simulink model "rtwdemo_sil_counter"  (Simulink 7.6)
settings: Solver=FixedStepDiscrete  StartTime=0.0  StopTime=10.0  FixedStep=Auto  RelTol=1e-3  SampleTimeConstraint=STIndependent
model workspace (MAT data in the model file):
  myUpper : Simulink.Parameter (value not decoded)
  myLower : Simulink.Parameter (value not decoded)
PostLoadFcn:
  | rtwdemo_overrides='{''SupportAbsoluteTime'',''LaunchReport'',''PassReuseOutputArgsAs''}';
  | rtwconfiguredemo(gcs,'noop',false,rtwdemo_overrides);
  | rtwdemo_cs=getActiveConfigSet(gcs);
  | setProp(rtwdemo_cs,'CustomSymbolStr','$R$N$M');
  | set_param(gcs,'dirty','off');
  | clear rtwdemo_overrides rtwdemo_cs
  | 
  | rtwdemo_sil_modelblock_data
undefined symbols (not defined in the file or in its folder): Increment
Description:
  | Example model reference component.
settings Model: Creator=The MathWorks Inc.  ExtModeAutoUpdateStatusClock=off
settings DataIOCC: LimitDataPoints=off  SaveFormat=StructureWithTime  SaveOutput=off  SaveTime=off  SignalLoggingName=logsOut
settings OptimizationCC: InlineParams=on  UseIntDivNetSlope=on  InlineInvariantSignals=on  EnhancedBackFolding=on  BooleansAsBitfields=on  PassReuseOutputArgsAs=Individual arguments  StateBitsets=on  DataBitsets=on  UseTempVars=on  ZeroExternalMemoryAtStartup=off  ZeroInternalMemoryAtStartup=off  NoFixptDivByZeroProtection=on  EfficientFloat2IntCast=on  OptimizeModelRefInitCode=on  LifeSpan=1  SimCompilerOptimization=On
settings DebuggingCC: MergeDetectMultiDrivingBlocksExec=error  CheckExecutionContextPreStartOutputMsg=on  CheckExecutionContextRuntimeOutputMsg=on  SolverPrmCheckMsg=none  UniqueDataStoreMsg=error  ModelReferenceSymbolNameMessage=none  StrictBusMsg=ErrorOnBusTreatedAsVector
settings HardwareCC: ProdIntDivRoundTo=Zero  ProdEndianess=LittleEndian  ProdHWDeviceType=Specified  TargetHWDeviceType=Generic->32-bit Embedded Processor
settings ModelReferenceCC: CheckModelReferenceTargetMessage=none  ModelReferencePassRootInputsByReference=off
settings RTWCC: SystemTargetFile=ert.tlc  TLCOptions=-p0 -aWarnNonSaturatedBlocks=0  TemplateMakefile=ert_default_tmf  Description=Real-Time Workshop Embedded Coder  GenerateReport=on  RTWVerbose=off  ProcessScript=ert_make_rtw_hook  IncludeHyperlinkInReport=on  GenerateTraceInfo=on  GenerateTraceReport=on  GenerateTraceReportSl=on  GenerateTraceReportSf=on  GenerateTraceReportEml=on
settings CodeAppCC: ForceParamTrailComments=on  IgnoreCustomStorageClasses=off  IgnoreTestpoints=on  SimulinkDataObjDesc=on  CustomSymbolStrGlobalVar=rt$N$M  CustomSymbolStrType=$N$M  CustomSymbolStrFcn=$N$M$F  CustomSymbolStrMacro=$N$M  InsertBlockDesc=on
settings ERTTargetCC: MultiwordLength=2048  GenerateSampleERTMain=on  IncludeMdlTerminateFcn=off  CombineSignalStateStructs=on  SupportAbsoluteTime=off  SupportNonFinite=off  SupportComplex=off  InlinedParameterPlacement=NonHierarchical  ERTCustomFileTemplate=example_file_process.tlc  ERTFilePackagingFormat=CompactWithDataFile  ConvertIfToSwitch=off

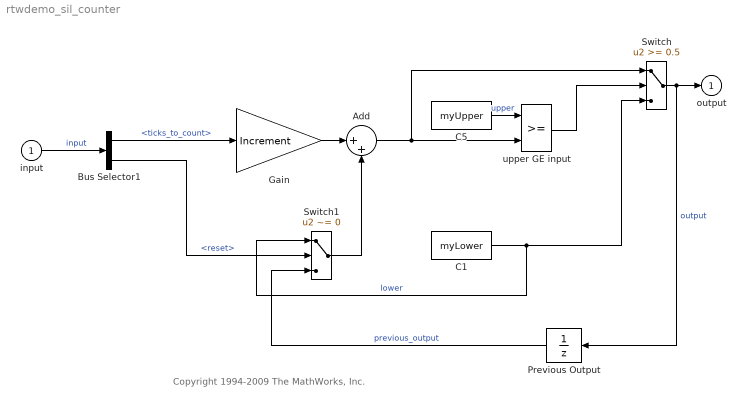
== system rtwdemo_sil_counter ==
  note: Copyright 1994-2009 The MathWorks, Inc.
  " input" : Inport  OutDataTypeStr=Bus: SilCounterBus  PortDimensions=1
  Add : Sum  Inputs=|++
  Bus Selector1 : BusSelector  OutputSignals=ticks_to_count,reset
  C1 : Constant  Value=myLower  OutDataTypeStr=uint8
  C5 : Constant  Value=myUpper  OutDataTypeStr=uint8
  Gain : Gain  Gain=Increment  ParamDataTypeStr=uint8  OutDataTypeStr=uint8
  Previous Output : UnitDelay  X0=50  SampleTime=-1
  Switch : Switch  Threshold=0.5  InputSameDT=on
  Switch1 : Switch  Criteria=u2 ~= 0  Threshold=0.5  InputSameDT=on
  upper GE input : RelationalOperator  Priority=0  InputSameDT=on
      settings: AttributesFormatString=\n
  output : Outport
  wires:
  Switch/1 -> output/1, Previous Output/1  "output"
  upper GE input/1 -> Switch/2
  " input"/1 -> Bus Selector1/1  "input"
  C5/1 -> upper GE input/1  "upper"
  Add/1 -> upper GE input/2, Switch/1
  Gain/1 -> Add/1
  C1/1 -> Switch/3, Switch1/1  "lower"
  Bus Selector1/1 -> Gain/1  "<ticks_to_count>"
  Bus Selector1/2 -> Switch1/2  "<reset>"
  Previous Output/1 -> Switch1/3  "previous_output"
  Switch1/1 -> Add/2
